simulink library "components_lib"  (Simulink 6.2)
undefined symbols (not defined in the file): A_ang_c, A_att_c, A_est, A_kalman, albedo_onboard_wrapper, B_ang_c, B_att_c, B_est, B_kalman, C_ang_c, C_att_c, C_est, C_i, C_kalman, C_p, Cd, D_ang_c, D_att_c, D_est, D_kalman, Dim, DiscIntNeverNeededParam, Hr, Hs, inerti, Ki, Kr, Ks, magnitude, otoquest, otoquest_with_pro, qmethod, rho, sat_temp_start, ss_proj3, sun_emu_angles2currents, sun_emu_vec2angles, Ts, vector_projection_onto_plane, w_mw_i, w_mw_init, zenith2ref
libraries: components_lib x163, simulink x44, albedo_lib x4, Accessories_lib x3, simulink_extras x2, discrete_bdot_filter x1
(part 4 of 5)

== system components_lib/Orbit and Ephemeris/Orbit and Magnetic field models/SGP4 position ==
  note: Other TLE
  note: Oersted TLE
  JD : Inport  Port=1  LatchInput=off
  Enable : EnablePort
  " S-Function" : S-Function  FunctionName=sgp4S
  Constant : Constant  Value=enable_oersted_tle
  Constant1 : Constant  Value=enable_other_tle
  Demux1 : Demux  Outputs=[3 3]
  Gain 1440 : Gain  Orientation=down  Gain=1440  SaturateOnIntegerOverflow=on
  Mux : Mux  Inputs=2
  Sum : Sum  Orientation=down  Inputs=-+|  SaturateOnIntegerOverflow=on  InputSameDT=on
  Sum1 : Sum  SaturateOnIntegerOverflow=on  InputSameDT=on
  Sum2 : Sum  SaturateOnIntegerOverflow=on  InputSameDT=on
  TLE and time initialization1 : Subsystem  mask{satname='Orsted', YYDDD=02039, JulianDay=2452275.5+40.69255057, xndt2o=0.00002748*0, xndd6o=0, bstar=0.00071190, xincl=96.4788, xnodeo=112.1945, eo=0.0148615, omegao=71.6037, xmo=290.1241, xno=14.43891950, ts=1}
      mask prompts: satname "Satellite Name:"; YYDDD "Epoch [YYDDD]:"; JulianDay "Epoch [JD]:"; xndt2o "MM dot:"; xndd6o "MM dot dot:"; bstar "Drag:"; xincl "Inclination [deg]:"; xnodeo "Right Ascension of Ascending Node [deg]:"; eo "Eccentricity [-]:"; omegao "Argument of Perigee [deg]:"; xmo "Mean Anomaly [deg]:"; xno "Mean Motion [rev/day]:"; ts "Sampling Time [sec]:"
      mask help:
      | Input TLE from the standard Two-Line Orbital Element Set Format
      | Satellite Name, Line 1 and 2.
      mask Display:
      | text(0.35,0.6,'Orbit');
      | text(0.33,0.5,'Model');
      | text(0.3,0.4,'Config');
  TLE and time initialization2 : Subsystem  mask{satname='Orsted', YYDDD=02039, JulianDay=2452275.5+40.69255057, xndt2o=0.00002748*0, xndd6o=0, bstar=0.00071190, xincl=96.4788, xnodeo=112.1945, eo=0.0148615, omegao=71.6037, xmo=290.1241, xno=14.43891950, ts=1}
      mask prompts: satname "Satellite Name:"; YYDDD "Epoch [YYDDD]:"; JulianDay "Epoch [JD]:"; xndt2o "MM dot:"; xndd6o "MM dot dot:"; bstar "Drag:"; xincl "Inclination [deg]:"; xnodeo "Right Ascension of Ascending Node [deg]:"; eo "Eccentricity [-]:"; omegao "Argument of Perigee [deg]:"; xmo "Mean Anomaly [deg]:"; xno "Mean Motion [rev/day]:"; ts "Sampling Time [sec]:"
      mask help:
      | Input TLE from the standard Two-Line Orbital Element Set Format
      | Satellite Name, Line 1 and 2.
      mask Display:
      | text(0.35,0.6,'Orbit');
      | text(0.33,0.5,'Model');
      | text(0.3,0.4,'Config');
  "km -> m" : Gain  Gain=1000  SaturateOnIntegerOverflow=on
  "km/s -> m/s" : Gain  Gain=1000  SaturateOnIntegerOverflow=on
  Position (I) : Outport  InitialOutput=0
  Velocity (I) : Outport  Port=2  InitialOutput=0
  wires:
  [Other_InitJD] -> Sum2/2
  [Oersted_InitJD] -> Sum2/1
  Sum1/1 -> Mux/2
  [Other_TLE] -> Sum1/2
  [Oersted_TLE] -> Sum1/1
  Constant1/1 -> TLE and time initialization2/1(Enable?)
  Constant/1 -> TLE and time initialization1/1(Enable?)
  Gain 1440/1 -> Mux/1
  Sum/1 -> Gain 1440/1
  Sum2/1 -> Sum/1
  Demux1/1 -> "km -> m"/1
  Demux1/2 -> "km/s -> m/s"/1
  " S-Function"/1 -> Demux1/1
  Mux/1 -> " S-Function"/1
  "km/s -> m/s"/1 -> Velocity (I)/1
  "km -> m"/1 -> Position (I)/1
  JD/1 -> Sum/2

== system components_lib/Sensor Emulation/Emulation of gyros/Amplification and ADC ==
  V_cont : Inport  Port=1  LatchInput=off
  Op amp gain [] : Gain  Gain=op_amp_gain
  Quantizer : Quantizer  QuantizationInterval=1/(2^12)
  Sum : Sum  Inputs=|+-
  Sum1 : Sum  Inputs=|++
  op_amp offset [mV] : Constant  Value=op_amp_offset
  V_discrete : Outport
  wires:
  Op amp gain []/1 -> Sum1/1
  Sum/1 -> Op amp gain []/1
  op_amp offset [mV]/1 -> Sum/2, Sum1/2
  V_cont/1 -> Sum/1
  Sum1/1 -> Quantizer/1
  Quantizer/1 -> V_discrete/1

== system components_lib/Sensor Emulation/Emulation of gyros/Gyro sensor block ==
  W(S) [rad/s] : Inport  Port=1  LatchInput=off
  Temperature [K] : Inport  Port=2  LatchInput=off
  Bias [degree/s] : Constant  Value=e_bias
  Drift(offset) [rad/s/K] : Constant  Value=e_drift_offset_model
  Drift(scale factor) [%/K] : Constant  Value=e_drift_scale_model
  "Missalignment correction factor Caculated in mask \"initialization commands\" based on the data supplied in the  missalignment parameter field" : Constant  Value=e_align_coor_factor
  Noise : RandomNumber  Variance=e_noise  Seed=e_noise_seed  SampleTime=0
  Offset  [mV] : Constant  Orientation=up  Value=offset_model
  Product1 : Product  SaturateOnIntegerOverflow=on
  Product2 : Product  Inputs=3  SaturateOnIntegerOverflow=on
  Product3 : Product  SaturateOnIntegerOverflow=on
  Product4 : Product  SaturateOnIntegerOverflow=on
  Scale error [%] : Constant  Value=e_scale
  Sum : Sum  Inputs=|++
  Sum1 : Sum  Inputs=++++++  SaturateOnIntegerOverflow=on
  Sum2 : Sum  Inputs=|+-
  Used for proper  adding of disturbances : Gain  Gain=[1 1 1 -1 -1 -1]
  Used for proper  adding of disturbances1 : Gain  Gain=[1 1 1 -1 -1 -1]
  convert percent to scale factor : Gain  Gain=0.01
  convert percent to scale factor1 : Gain  Gain=0.01
  scale factor : Gain  Gain=scale_model
  temp must be deviation from 25 degree C : Constant  Orientation=up  Value=298.15
  W_sens(S) [mV] : Outport
  wires:
  Noise/1 -> Sum1/4
  Sum1/1 -> Used for proper  adding of disturbances1/1
  W(S) [rad/s]/1 -> Used for proper  adding of disturbances/1
  Product1/1 -> Sum1/1
  Product4/1 -> Sum1/6
  Temperature [K]/1 -> Sum2/1
  temp must be deviation from 25 degree C/1 -> Sum2/2
  Drift(scale factor) [%/K]/1 -> convert percent to scale factor1/1
  Drift(offset) [rad/s/K]/1 -> Product4/2
  convert percent to scale factor1/1 -> Product2/2
  Product2/1 -> Sum1/5
  Bias [degree/s]/1 -> Sum1/3
  convert percent to scale factor/1 -> Product3/1
  Product3/1 -> Sum1/2
  Scale error [%]/1 -> convert percent to scale factor/1
  Used for proper  adding of disturbances/1 -> Product2/1, Product1/2, Product3/2
  "Missalignment correction factor Caculated in mask \"initialization commands\" based on the data supplied in the  missalignment parameter field"/1 -> Product1/1
  Sum2/1 -> Product4/1, Product2/3
  Offset  [mV]/1 -> Sum/2
  Sum/1 -> W_sens(S) [mV]/1
  scale factor/1 -> Sum/1
  Used for proper  adding of disturbances1/1 -> scale factor/1

== system components_lib/Sensor Emulation/Emulation of magnetometer/Amplification and ADC ==
  V_cont : Inport  Port=1  LatchInput=off
  Op amp gain [] : Gain  Gain=op_amp_gain
  Quantizer : Quantizer  QuantizationInterval=1/(2^12)
  Sum1 : Sum  Inputs=|++
  op_amp offset [mV] : Constant  Value=op_amp_offset
  V_discrete : Outport
  wires:
  Quantizer/1 -> V_discrete/1
  Op amp gain []/1 -> Sum1/1
  op_amp offset [mV]/1 -> Sum1/2
  V_cont/1 -> Op amp gain []/1
  Sum1/1 -> Quantizer/1

== system components_lib/Sensor Emulation/Emulation of magnetometer/magnetometer sensor block ==
  B(I) : Inport  Port=1  LatchInput=off
  q(I->S) : Inport  Port=2  LatchInput=off
  Temperature  [K] : Inport  Port=3  LatchInput=off
  Drift(sensitivity) [ppm/K] : Constant  Value=e_drift_sens_model
  "Misalignment correction factor Caculated in mask \"initialization commands\" based on the data supplied in the  misalignment parameter field" : Constant  Value=e_align_coor_factor
  Noise : RandomNumber  Variance=e_noise  Seed=e_noise_seed  SampleTime=0
  Offset  [mV] : Constant  Orientation=up  Value=0
  Scale error : Product  SaturateOnIntegerOverflow=on
  Scale error [%] : Constant  Value=e_scale
  Sensitivity : Gain  Gain=sens_model
  Sum : Sum  Inputs=|++
  Sum1 : Sum  Inputs=++++  SaturateOnIntegerOverflow=on
  Sum2 : Sum  Inputs=|+-
  V*Gauss->Gauss : Gain  Gain=v_supply_model
  Vector rotation by q1 : Subsystem  AncestorBlock=components_lib/Math utilities/Vector operations/Vector rotation by q
  alignment corection  (both orthogonality and  misalignment) : Product  Multiplication=Matrix(*)  SaturateOnIntegerOverflow=on
  convert percent to scale factor : Gain  Gain=0.01
  convert ppm to scale factor : Gain  Gain=10e-6
  sensitivity  temperature  drift [Gauss] : Product  Inputs=3  SaturateOnIntegerOverflow=on
  temp must be deviation from 25 degree C : Constant  Orientation=up  Value=298.15
  Voltage  [mV] : Outport
  wires:
  Sum1/1 -> Sensitivity/1
  Temperature  [K]/1 -> Sum2/1
  temp must be deviation from 25 degree C/1 -> Sum2/2
  q(I->S)/1 -> Vector rotation by q1/1(q)
  "Misalignment correction factor Caculated in mask \"initialization commands\" based on the data supplied in the  misalignment parameter field"/1 -> alignment corection  (both orthogonality and  misalignment)/1
  alignment corection  (both orthogonality and  misalignment)/1 -> sensitivity  temperature  drift [Gauss]/1, Sum1/2, Scale error/2
  Drift(sensitivity) [ppm/K]/1 -> convert ppm to scale factor/1
  convert ppm to scale factor/1 -> sensitivity  temperature  drift [Gauss]/2
  Sum2/1 -> sensitivity  temperature  drift [Gauss]/3
  Vector rotation by q1/1(q'Vq) -> alignment corection  (both orthogonality and  misalignment)/2  "B(S)"
  Sum/1 -> Voltage  [mV]/1
  Sensitivity/1 -> V*Gauss->Gauss/1
  Offset  [mV]/1 -> Sum/2
  V*Gauss->Gauss/1 -> Sum/1
  B(I)/1 -> Vector rotation by q1/2(V)
  sensitivity  temperature  drift [Gauss]/1 -> Sum1/3
  convert percent to scale factor/1 -> Scale error/1
  Scale error/1 -> Sum1/1
  Scale error [%]/1 -> convert percent to scale factor/1
  Noise/1 -> Sum1/4

== system components_lib/Sensor Emulation/Sun sensors/Amplification and ADC ==
  Currents [mA] : Inport  Port=1  LatchInput=off
  Op amp gain : Gain  Gain=op_amp_gain
  Quantizer : Quantizer  QuantizationInterval=1/(2^12)
  Sum1 : Sum  Inputs=|++
  op_amp offset [mV] : Constant  Value=op_amp_offset
  I_ADC [mA] : Outport
  wires:
  Sum1/1 -> Quantizer/1
  Quantizer/1 -> I_ADC [mA]/1
  Op amp gain/1 -> Sum1/1
  op_amp offset [mV]/1 -> Sum1/2
  Currents [mA]/1 -> Op amp gain/1

== system components_lib/Sensor Emulation/Sun sensors/Frame conversion ==
  note: Sun vector
      | from sun to sat
      | in ECI
  Sun pos. R_s(I) : Inport  Port=1  LatchInput=off
  S/C pos. R_sa(I) : Inport  Port=2  LatchInput=off
  q(I->S) : Inport  Port=3  LatchInput=off
  q(I->E) : Inport  Port=4  LatchInput=off
  Quaternion inverter : components_lib/Math utilities/Quaternion operations/Quaternion inverter
  Rotation of q1 by q2 : components_lib/Math utilities/Quaternion operations/Rotation of q1 by q2
  Sum : Sum  Inputs=|+-
  Vector rotation by q : components_lib/Math utilities/Quaternion operations/Vector rotation by q
  Vector rotation by q3 : components_lib/Math utilities/Quaternion operations/Vector rotation by q
  "Zenith to nadir " : Gain  Gain=-1
  Sun pos. R_s(S) : Outport
  Nadir(E) : Outport  Port=2
  q(S->E) : Outport  Port=3
  wires:
  Sum/1 -> Vector rotation by q3/2
  Sun pos. R_s(I)/1 -> Sum/1
  Rotation of q1 by q2/1 -> q(S->E)/1
  Quaternion inverter/1 -> Rotation of q1 by q2/1
  q(I->S)/1 -> Quaternion inverter/1, Vector rotation by q3/1
  q(I->E)/1 -> Rotation of q1 by q2/2, Vector rotation by q/1
  "Zenith to nadir "/1 -> Nadir(E)/1
  S/C pos. R_sa(I)/1 -> Sum/2, Vector rotation by q/2
  Vector rotation by q/1 -> "Zenith to nadir "/1
  Vector rotation by q3/1 -> Sun pos. R_s(S)/1

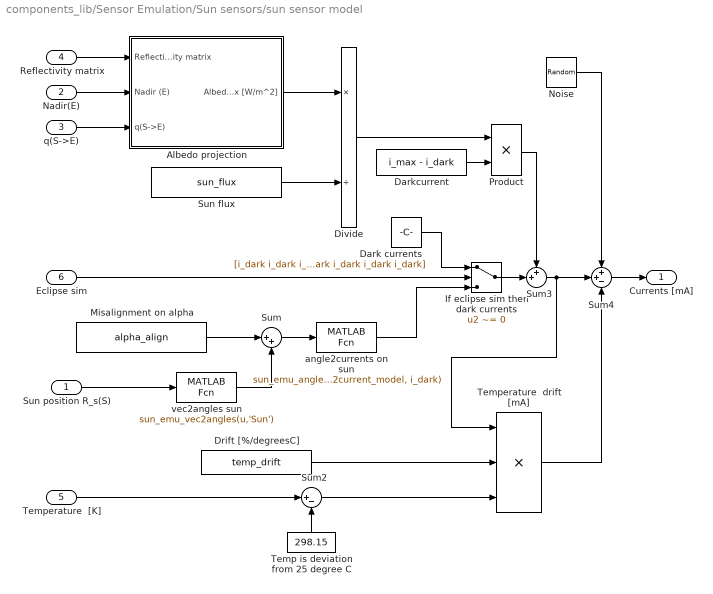
== system components_lib/Sensor Emulation/Sun sensors/sun sensor model ==
  Sun position R_s(S) : Inport  Port=1  LatchInput=off
  Nadir(E) : Inport  Port=2  LatchInput=off
  q(S->E) : Inport  Port=3  LatchInput=off
  Reflectivity matrix : Inport  Port=4  LatchInput=off
  Temperature  [K] : Inport  Port=5  LatchInput=off
  Eclipse sim : Inport  Port=6  PortDimensions=1  LatchInput=off
  Albedo projection : Subsystem
  Dark currents : Constant  Value=[i_dark i_dark i_dark i_dark i_dark i_dark]
  Darkcurrent : Constant  Value=i_max - i_dark
  Divide : Product  Inputs=*/  OutScaling=2^-10
  Drift [%/degreesC] : Constant  Value=temp_drift
  If eclipse sim then dark currents : Switch  Criteria=u2 ~= 0
  Misalignment on alpha : Constant  Value=alpha_align
  Noise : RandomNumber  Variance=sigma_noise^2  Seed=noise_seed  SampleTime=0
  Product : Product  RndMeth=Zero
  Sum : Sum  Inputs=|++
  Sum2 : Sum  Inputs=|+-
  Sum3 : Sum  Inputs=++|
  Sum4 : Sum  Inputs=++-
  Sun flux : Constant  Value=sun_flux
  Temp is deviation from 25 degree C : Constant  Orientation=up  Value=298.15
  Temperature  drift [mA] : Product  Inputs=3  SaturateOnIntegerOverflow=on
  angle2currents on sun : MATLABFcn  MATLABFcn=sun_emu_angles2currents(u,angle2current_model, i_dark)
  vec2angles sun : MATLABFcn  MATLABFcn=sun_emu_vec2angles(u,'Sun')
  Currents [mA] : Outport
  wires:
  If eclipse sim then dark currents/1 -> Sum3/2
  angle2currents on sun/1 -> If eclipse sim then dark currents/3
  Eclipse sim/1 -> If eclipse sim then dark currents/2
  Dark currents/1 -> If eclipse sim then dark currents/1
  Sum4/1 -> Currents [mA]/1
  Temperature  drift [mA]/1 -> Sum4/3
  Sum3/1 -> Sum4/2, Temperature  drift [mA]/1
  Product/1 -> Sum3/1
  Temperature  [K]/1 -> Sum2/1
  Noise/1 -> Sum4/1
  Albedo projection/1(Albedo flux [W/m^2]) -> Divide/1
  Nadir(E)/1 -> Albedo projection/2(Nadir (E))
  q(S->E)/1 -> Albedo projection/3(q(S->E))
  Reflectivity matrix/1 -> Albedo projection/1(Reflectivity matrix)
  Darkcurrent/1 -> Product/2
  Temp is deviation from 25 degree C/1 -> Sum2/2
  Misalignment on alpha/1 -> Sum/1
  vec2angles sun/1 -> Sum/2
  Sum/1 -> angle2currents on sun/1
  Sum2/1 -> Temperature  drift [mA]/3
  Drift [%/degreesC]/1 -> Temperature  drift [mA]/2
  Sun position R_s(S)/1 -> vec2angles sun/1
  Sun flux/1 -> Divide/2
  Divide/1 -> Product/1

== system components_lib/ACS/Controllers/Desaturation controller/Trigger ==
  B_unit(s) : Inport  Port=1  PortDimensions=3  LatchInput=off
  h_err : Inport  Port=2  LatchInput=off
  Dot Product2 : simulink/Math Operations/Dot Product  InputSameDT=on  OutDataType=sfix(16)  OutScaling=2^-10  DoSatur=off
  Dot Product3 : simulink/Math Operations/Dot Product  InputSameDT=on  OutDataType=sfix(16)  OutScaling=2^-10  DoSatur=off
  Math Function1 : Math  Operator=sqrt  SaturateOnIntegerOverflow=on
  Math Function3 : Math  Operator=sqrt  SaturateOnIntegerOverflow=on
  Relay : Subsystem
  Saturation : Saturate  UpperLimit=inf  LowerLimit=2*sin(deg2rad(2))*h_bias
  Sum1 : Sum  Inputs=|+-
  angular momentum bias1 : Constant  Value=sin(deg2rad(2))*h_bias
  angular momentum bias3 : Constant  Value=2*5.48e-5
  angular momentum bias4 : Constant  Value=h_bias
  cross_product : components_lib/Math utilities/Vector operations/cross_product_no_fnc
  mag B div1 : Product  Inputs=*/  OutScaling=2^-10
  mg B div4 : Product  OutScaling=2^-10
  switch : Outport
  wires:
  angular momentum bias3/1 -> Sum1/2
  Relay/1(Switch) -> switch/1
  angular momentum bias4/1 -> mg B div4/2
  mg B div4/1 -> Sum1/1
  Dot Product2/1 -> Math Function3/1
  Dot Product3/1 -> Math Function1/1
  Math Function1/1 -> mag B div1/2
  Sum1/1 -> Saturation/1
  mag B div1/1 -> mg B div4/1  "sin(a)"
  h_err/1 -> Dot Product3/1, Dot Product3/2, cross_product/1
  B_unit(s)/1 -> cross_product/2
  cross_product/1 -> Dot Product2/1, Dot Product2/2
  Math Function3/1 -> mag B div1/1, Relay/1(||Herr x B_unit||)
  angular momentum bias1/1 -> Relay/3(lower limet)
  Saturation/1 -> Relay/2(upper limet)

== system components_lib/ACS/Controllers/Desaturation controller/m_mt to v_mt conversion ==
  m_mt : Inport  Port=1  LatchInput=off
  T_meas : Inport  Port=2  LatchInput=off
  Demux : Demux  Outputs=3
  Gain : Gain  Gain=1/(n_mt(1)*A_mt(1))
  Gain1 : Gain  Gain=1/(n_mt(2)*A_mt(2))
  Gain2 : Gain  Gain=1/(n_mt(3)*A_mt(3))
  Mux : Mux  Inputs=3
  Resistance for mt on x-axis : Subsystem  mask{A_wire_mt=(pi/4)*0.0002^2, sigma_0_mt=1.7e-8, alpha_0_mt=3.9e-3, T_0_mt=293}
      mask prompts: A_wire_mt "Wire cross sectional area"; sigma_0_mt "Wire resistivity"; alpha_0_mt "Wire resistivity temp. coef."; T_0_mt "Wire resistivity base temp."
  Resistance for mt on y-axis : Subsystem  mask{A_wire_mt=(pi/4)*0.0002^2, sigma_0_mt=1.7e-8, alpha_0_mt=3.9e-3, T_0_mt=293}
      mask prompts: A_wire_mt "Wire cross sectional area"; sigma_0_mt "Wire resistivity"; alpha_0_mt "Wire resistivity temp. coef."; T_0_mt "Wire resistivity base temp."
  Resistance for mt on z-axis : Subsystem  mask{A_wire_mt=(pi/4)*0.0002^2, sigma_0_mt=1.7e-8, alpha_0_mt=3.9e-3, T_0_mt=293}
      mask prompts: A_wire_mt "Wire cross sectional area"; sigma_0_mt "Wire resistivity"; alpha_0_mt "Wire resistivity temp. coef."; T_0_mt "Wire resistivity base temp."
  electromechanis transfer funtion for mt_x : Subsystem
  "electromechanis transfer funtion for mt_y " : Subsystem
  "electromechanis transfer funtion for mt_z " : Subsystem
  i_mt : Scope  NumInputPorts=3
      settings: YMin=-5~-5~-5  YMax=5~5~5  SaveName=ScopeData8
  v_mt : Outport
  wires:
  Demux/3 -> Gain2/1
  Demux/2 -> Gain1/1
  Demux/1 -> Gain/1
  Gain/1 -> electromechanis transfer funtion for mt_x/1(i_mt), i_mt/1
  Gain1/1 -> "electromechanis transfer funtion for mt_y "/1(i_mt), i_mt/2
  Gain2/1 -> "electromechanis transfer funtion for mt_z "/1(i_mt), i_mt/3
  m_mt/1 -> Demux/1
  "electromechanis transfer funtion for mt_y "/1(v_mt) -> Mux/2
  "electromechanis transfer funtion for mt_z "/1(v_mt) -> Mux/3
  Resistance for mt on x-axis/1(R(T)) -> electromechanis transfer funtion for mt_x/2(R(T))
  Resistance for mt on y-axis/1(R(T)) -> "electromechanis transfer funtion for mt_y "/2(R(T))
  Resistance for mt on z-axis/1(R(T)) -> "electromechanis transfer funtion for mt_z "/2(R(T))
  T_meas/1 -> Resistance for mt on y-axis/1(T), Resistance for mt on x-axis/1(T), Resistance for mt on z-axis/1(T)
  electromechanis transfer funtion for mt_x/1(v_mt) -> Mux/1
  Mux/1 -> v_mt/1

== system components_lib/ACS/Controllers/Detumble controller/Continous B-dot controller ==
  B(S) : Inport  Port=1  LatchInput=off
  Gain : Gain  Gain=w_c
  Gain1 : Gain  Gain=-C_cont
  Integrator : Integrator  Orientation=left
  Sum : Sum  Inputs=|+-
  m_mt(S) : Outport
  wires:
  B(S)/1 -> Sum/1
  Sum/1 -> Gain/1
  Gain/1 -> Gain1/1, Integrator/1
  Integrator/1 -> Sum/2
  Gain1/1 -> m_mt(S)/1

== system components_lib/ACS/Controllers/Detumble controller/Discrete B-dot controller ==
  B(S) : Inport  Port=1  LatchInput=off
  Clock : Clock
  Discrete B-dot filter : discrete_bdot_filter/Discrete B-dot filter
  Gain1 : Gain  Gain=-C_disc
  If : If  IfExpression=u1 > 2
  If1 : If  IfExpression=u1 < 4
  If2 : If  IfExpression=u1 < 2
  Subsystem1 : Subsystem  AncestorBlock=attitude_control_lib/Attitude Control/B-dot controller disc/Subsystem2
  Subsystem2 : Subsystem  AncestorBlock=attitude_control_lib/Attitude Control/B-dot controller disc/Subsystem2
  Subsystem3 : Subsystem  AncestorBlock=attitude_control_lib/Attitude Control/B-dot controller disc/Subsystem2
  mod 10 : MATLABFcn  MATLABFcn=mod(u(1),4)
  m_mt(s) : Outport
  wires:
  Discrete B-dot filter/1 -> Gain1/1
  If1/1 -> Subsystem3/Action
  Subsystem2/1(Out1) -> m_mt(s)/1
  B(S)/1 -> Subsystem1/1(In1)
  Subsystem3/1(Out1) -> Subsystem2/1(In1)
  Gain1/1 -> Subsystem3/1(In1)
  Subsystem1/1(Out1) -> Discrete B-dot filter/1
  Clock/1 -> mod 10/1
  mod 10/1 -> If2/1, If1/1, If/1
  If2/1 -> Subsystem1/Action
  If/1 -> Subsystem2/Action

== system components_lib/ACS/Controllers/Detumble controller/Magnetic field I to S ==
  q(I->S) : Inport  Port=1  LatchInput=off
  B(I) : Inport  Port=2  LatchInput=off
  Gauss to Tesla : Gain  Gain=1e-4
  Vector rotation by q1 : components_lib/Math utilities/Quaternion operations/Vector rotation by q
  B(S) : Outport
  wires:
  B(I)/1 -> Vector rotation by q1/2
  Gauss to Tesla/1 -> B(S)/1
  Vector rotation by q1/1 -> Gauss to Tesla/1
  q(I->S)/1 -> Vector rotation by q1/1

== system components_lib/ACS/Controllers/Detumble controller/enable/disable continous controller ==
  In1 : Inport  Port=1  LatchInput=off
  Action Port : ActionPort
  Out1 : Outport
  wires:
  In1/1 -> Out1/1

== system components_lib/ACS/Controllers/Detumble controller/enable/disable discrete controller ==
  In1 : Inport  Port=1  LatchInput=off
  Action Port : ActionPort
  Out1 : Outport
  wires:
  In1/1 -> Out1/1

== system components_lib/ADS/On-board model/ADS on-board models/Albedo model onboard ==
  "Earth -> Sun vector (ECEF)" : Inport  Port=1  LatchInput=off
  Zenith vector (ECEF) : Inport  Port=2  LatchInput=off
  q(I->S) : Inport  Port=3  LatchInput=off
  q(I->E) : Inport  Port=4  LatchInput=off
  On : Constant  Orientation=down  Value=enable
  On1 : Constant  Orientation=down  Value=~enable
  Sum : Sum  Inputs=|++
  cos dependent albedo : Subsystem
  fov matrix albedo : Subsystem
  Albedo vector (I) : Outport
  wires:
  On1/1 -> cos dependent albedo/Enable
  fov matrix albedo/1(Albedo vector (I)) -> Sum/2
  cos dependent albedo/1(Albedo vector (I)) -> Sum/1
  On/1 -> fov matrix albedo/Enable
  Zenith vector (ECEF)/1 -> fov matrix albedo/1(Zenith vector (ECEF)), cos dependent albedo/2(Zenith vector (ECEF))
  "Earth -> Sun vector (ECEF)"/1 -> fov matrix albedo/2("Earth -> Sun vector (ECEF)"), cos dependent albedo/1("Earth -> Sun vector (ECEF)")
  q(I->E)/1 -> fov matrix albedo/4(q(I->E))
  q(I->S)/1 -> fov matrix albedo/3(q(I->S))
  Sum/1 -> Albedo vector (I)/1

== system components_lib/ADS/On-board model/Albedo model onboard/cos dependent albedo ==
  note: Projection onto
      | the zenith vector
  "Earth -> Sun vector (ECEF)" : Inport  Port=1  LatchInput=off
  Zenith vector (ECEF) : Inport  Port=2  LatchInput=off
  Enable : EnablePort  StatesWhenEnabling=reset
  Abs : Abs
  Dot Product : simulink/Math Operations/Dot Product  InputSameDT=on  OutDataType=sfix(16)  OutScaling=2^-10  DoSatur=off
  Mean solar flux (1366.9 [W/m^2]) : Constant  Value=sun_flux
  Product : Product  RndMeth=Zero
  Product1 : Product  RndMeth=Zero
  Product2 : Product  RndMeth=Zero
  Sun vector  to unit vector : components_lib/Math utilities/Vector operations/to unit vector
  Zentih vector to unit vector : components_lib/Math utilities/Vector operations/to unit vector
  "zenith2ref(u, mrm)" : MATLABFcn  MATLABFcn=zenith2ref(u, mrm)*2
  Albedo vector (I) : Outport
  wires:
  Product2/1 -> Albedo vector (I)/1
  Product1/1 -> Product2/1
  Abs/1 -> Product1/1
  Dot Product/1 -> Abs/1
  Sun vector  to unit vector/1 -> Product/1
  Mean solar flux (1366.9 [W/m^2])/1 -> Product/2
  Product/1 -> Dot Product/1
  "zenith2ref(u, mrm)"/1 -> Product1/2
  Zentih vector to unit vector/1 -> Product2/2, "zenith2ref(u, mrm)"/1, Dot Product/2
  "Earth -> Sun vector (ECEF)"/1 -> Sun vector  to unit vector/1
  Zenith vector (ECEF)/1 -> Zentih vector to unit vector/1

== system components_lib/ADS/On-board model/Albedo model onboard/fov matrix albedo ==
  Zenith vector (ECEF) : Inport  Port=1  LatchInput=off
  "Earth -> Sun vector (ECEF)" : Inport  Port=2  LatchInput=off
  q(I->S) : Inport  Port=3  LatchInput=off
  q(I->E) : Inport  Port=4  LatchInput=off
  Enable : EnablePort  StatesWhenEnabling=reset
  Albedo projection : components_lib/ADS/On-board Sensor model/Albedo projection
  Demux : Demux  Outputs=2
  Earth Albedo Model : Subsystem  TreatAsAtomicUnit=on  mask(Earth Albedo Model){eprdata=load('lib/space_environment_emulation/albedo/toolbox/epr_data/2003/ga030101-031231'), redfac=10, Ts=1, enable=on}
      mask prompts: eprdata "Reflectivity Data (EPR Struct):"; redfac "Reduction factor:"; Ts "Sample Time (-1 for inherited):"
      mask help: Calculate Earth Albedo using static data from the EP/TOMS spacecraft.
      mask init:
      | global sy;
      | global sx;
      | sy = round(180/redfac);
      | sx = round(288/redfac);
      mask Help:
      | <b>Input</b><br>
      | Sat: Vector to satellite in ECEF [m]<br>
      | Sun: Vector to the Sun in ECEF [m]<p>
      | <b>Parameters</b><br>
      | Reflectivity Data (EPR Struct): TOMS Reflectivity data [E.U].<br>
      | Reduction factor: Reduce data resolution by this factor.<br>
      | Sample Time (-1 for inherited): Sample Time [s]. The block cannot inherit continuous sample time.<br>
      | Enable: Enable or disable albedo calculation<p>
      | <b>Output</b><br>
      | Albedo: Fraction of solar irradiance received on the satellite. The incoming solar irradiance is 1366.5 W/m^2<p>
      mask CallbackString: |||enable = strcmp(get_param(gcb,'enable'),'on');
      mask Display:
      | image(imread('private/albedoicon.png'));
      | port_label('output', 1, 'Albedo');
      | port_label('input', 1, 'Sat');
      | port_label('input', 2, 'Sun');
  Quaternion inverter1 : components_lib/Math utilities/Quaternion operations/Quaternion inverter
  Rotation of q1 by q2 : components_lib/Math utilities/Quaternion operations/Rotation of q1 by q2
  Sum : Sum  Inputs=|+-
  Vector rotation by q4 : components_lib/Math utilities/Quaternion operations/Vector rotation by q
  "Zenith to nadir " : Gain  Gain=-1
  Albedo vector (I) : Outport
  wires:
  "Earth -> Sun vector (ECEF)"/1 -> Earth Albedo Model/2(r_sun_ecef)
  Zenith vector (ECEF)/1 -> "Zenith to nadir "/1, Earth Albedo Model/1(r_sat_ecef)
  Vector rotation by q4/1 -> Albedo vector (I)/1
  q(I->E)/1 -> Rotation of q1 by q2/2
  q(I->S)/1 -> Quaternion inverter1/1
  Earth Albedo Model/1(a) -> Albedo projection/1
  "Zenith to nadir "/1 -> Albedo projection/2
  Quaternion inverter1/1 -> Rotation of q1 by q2/1, Vector rotation by q4/1
  Rotation of q1 by q2/1 -> Albedo projection/3
  Albedo projection/1 -> Demux/1
  Demux/1 -> Sum/1
  Demux/2 -> Sum/2
  Sum/1 -> Vector rotation by q4/2

== system components_lib/ADS/On-board model/Ephemeris on-board/ECEF ==
  t(JD) : Inport  Port=1  LatchInput=off
  eci2ecef : MATLABFcn  MATLABFcn=eci2ecef  OutputDimensions=4
  q(I->E) : Outport
  wires:
  eci2ecef/1 -> q(I->E)/1
  t(JD)/1 -> eci2ecef/1

== system components_lib/ADS/On-board model/Ephemeris on-board/Sun Position ==
  t(JD) : Inport  Port=1  LatchInput=off
  Sun R in ECI : MATLABFcn  MATLABFcn=sun  OutputDimensions=3
  R_s(I) : Outport
  wires:
  t(JD)/1 -> Sun R in ECI/1
  Sun R in ECI/1 -> R_s(I)/1

== system components_lib/ADS/On-board model/Gyros/Combine the angular rate  from the 6 gyros to angular  rate in S-frame ==
  W_meas 6 gyros : Inport  Port=1  LatchInput=off
  Demux : Demux  Outputs=6
  Gain1 : Gain  Gain=0.5
  Mux : Mux  Inputs=3
  Sum : Sum  Inputs=|+-
  Sum5 : Sum  Inputs=|+-
  Sum6 : Sum  Inputs=|+-
  W_meas (S) : Outport
  wires:
  Gain1/1 -> W_meas (S)/1
  W_meas 6 gyros/1 -> Demux/1
  Mux/1 -> Gain1/1
  Sum6/1 -> Mux/3
  Sum5/1 -> Mux/2
  Sum/1 -> Mux/1
  Demux/6 -> Sum6/2
  Demux/3 -> Sum6/1
  Demux/5 -> Sum5/2
  Demux/2 -> Sum5/1
  Demux/4 -> Sum/2
  Demux/1 -> Sum/1

== system components_lib/ADS/On-board model/Orbit and Magnetic field models/TLE and time initialization1 ==
  Enable? : Inport  Port=1  LatchInput=off
  Create TLE and JD : Subsystem  TreatAsAtomicUnit=on
  Oersted_InitJD : Outport
  Oersted_TLE : Outport  Port=2
  wires:
  Enable?/1 -> Create TLE and JD/Enable
  Create TLE and JD/2("TLE ") -> Oersted_TLE/1
  Create TLE and JD/1(Init JD) -> Oersted_InitJD/1

== system components_lib/ADS/On-board model/Orbit and Magnetic field models/TLE and time initialization3 ==
  Enable? : Inport  Port=1  LatchInput=off
  Create TLE and JD : Subsystem  TreatAsAtomicUnit=on
  Other_InitJD : Outport
  Other_TLE : Outport  Port=2
  wires:
  Enable?/1 -> Create TLE and JD/Enable
  Create TLE and JD/2("TLE ") -> Other_TLE/1
  Create TLE and JD/1(Init JD) -> Other_InitJD/1

== system components_lib/Disturbances/Exposed area/Shadow Area/Subsystem ==
  x : Inport  Port=1  LatchInput=off
  Dot Product13 : simulink/Math Operations/Dot Product  InputSameDT=on  OutDataType=sfix(16)  OutScaling=2^-10  DoSatur=off
  inv9 : Math  Operator=sqrt  SaturateOnIntegerOverflow=on
  norm(x) : Outport
  wires:
  inv9/1 -> norm(x)/1
  Dot Product13/1 -> inv9/1
  x/1 -> Dot Product13/2, Dot Product13/1  "pxp"

== system components_lib/Disturbances/Exposed area/Shadow Area/Subsystem1 ==
  x : Inport  Port=1  LatchInput=off
  Dot Product13 : simulink/Math Operations/Dot Product  InputSameDT=on  OutDataType=sfix(16)  OutScaling=2^-10  DoSatur=off
  inv9 : Math  Operator=sqrt  SaturateOnIntegerOverflow=on
  norm(x) : Outport
  wires:
  x/1 -> Dot Product13/1, Dot Product13/2  "pxp"
  Dot Product13/1 -> inv9/1
  inv9/1 -> norm(x)/1

== system components_lib/Disturbances/Exposed area/Shadow Area/Subsystem2 ==
  x : Inport  Port=1  LatchInput=off
  Dot Product13 : simulink/Math Operations/Dot Product  InputSameDT=on  OutDataType=sfix(16)  OutScaling=2^-10  DoSatur=off
  inv9 : Math  Operator=sqrt  SaturateOnIntegerOverflow=on
  norm(x) : Outport
  wires:
  inv9/1 -> norm(x)/1
  Dot Product13/1 -> inv9/1
  x/1 -> Dot Product13/2, Dot Product13/1  "pxp"

== system components_lib/Disturbances/Exposed area/Shadow Area/Subsystem3 ==
  x : Inport  Port=1  LatchInput=off
  Dot Product13 : simulink/Math Operations/Dot Product  InputSameDT=on  OutDataType=sfix(16)  OutScaling=2^-10  DoSatur=off
  inv9 : Math  Operator=sqrt  SaturateOnIntegerOverflow=on
  norm(x) : Outport
  wires:
  inv9/1 -> norm(x)/1
  Dot Product13/1 -> inv9/1
  x/1 -> Dot Product13/2, Dot Product13/1  "pxp"

== system components_lib/Disturbances/Gravity/Gravity Gradient Torque/  ==
  q(C->SC) : Inport  Port=1  LatchInput=off
  "q(I -> SC)" : Inport  Port=2  LatchInput=off
  R_sc(I) : Inport  Port=3  LatchInput=off
  Reverse quaternion rotation : components_lib/Math utilities/Quaternion operations/Reverse quaternion rotation
  Rotation of q1 by q2 : components_lib/Math utilities/Quaternion operations/Rotation of q1 by q2
  Vector rotation by q : components_lib/Math utilities/Quaternion operations/Vector rotation by q
  to unit vector : components_lib/Math utilities/Vector operations/to unit vector
  R_sc(C) : Outport
  wires:
  Vector rotation by q/1 -> R_sc(C)/1
  to unit vector/1 -> Vector rotation by q/2
  Rotation of q1 by q2/1 -> Vector rotation by q/1
  R_sc(I)/1 -> to unit vector/1
  Reverse quaternion rotation/1 -> Rotation of q1 by q2/2
  q(C->SC)/1 -> Reverse quaternion rotation/1
  "q(I -> SC)"/1 -> Rotation of q1 by q2/1

== system components_lib/Math utilities/Quaternion operations/Reverse quaternion rotation/Quaternion inverter ==
  q : Inport  Port=1  LatchInput=off
  Demux : Demux
  Demux1 : Demux  Outputs=3
  Gain : Gain  Gain=-1  SaturateOnIntegerOverflow=on
  Mux : Mux
  Mux1 : Mux  Inputs=3
  q^-1 : Outport
  wires:
  Gain/1 -> Demux1/1
  Demux1/3 -> Mux/3
  Demux1/2 -> Mux/2
  Demux1/1 -> Mux/1
  Mux1/1 -> Gain/1
  Demux/3 -> Mux1/3
  Demux/2 -> Mux1/2
  Demux/1 -> Mux1/1
  Demux/4 -> Mux/4
  Mux/1 -> q^-1/1
  q/1 -> Demux/1

== system components_lib/Math utilities/Quaternion operations/Vector rotation by q/Quaternion inverter ==
  q : Inport  Port=1  LatchInput=off
  Demux : Demux
  Demux1 : Demux  Outputs=3
  Gain : Gain  Gain=-1  SaturateOnIntegerOverflow=on
  Mux : Mux
  Mux1 : Mux  Inputs=3
  q^-1 : Outport
  wires:
  Gain/1 -> Demux1/1
  Demux1/3 -> Mux/3
  Demux1/2 -> Mux/2
  Demux1/1 -> Mux/1
  Mux1/1 -> Gain/1
  Demux/3 -> Mux1/3
  Demux/2 -> Mux1/2
  Demux/1 -> Mux1/1
  Demux/4 -> Mux/4
  Mux/1 -> q^-1/1
  q/1 -> Demux/1

== system components_lib/Math utilities/Vector operations/Vector rotation by q/Quaternion inverter ==
  q : Inport  Port=1  LatchInput=off
  Demux : Demux
  Demux1 : Demux  Outputs=3
  Gain : Gain  Gain=-1  SaturateOnIntegerOverflow=on
  Mux : Mux
  Mux1 : Mux  Inputs=3
  q^-1 : Outport
  wires:
  Gain/1 -> Demux1/1
  Demux1/3 -> Mux/3
  Demux1/2 -> Mux/2
  Demux1/1 -> Mux/1
  Mux1/1 -> Gain/1
  Demux/3 -> Mux1/3
  Demux/2 -> Mux1/2
  Demux/1 -> Mux1/1
  Demux/4 -> Mux/4
  Mux/1 -> q^-1/1
  q/1 -> Demux/1

== system components_lib/Orbit and Ephemeris/Orbit and Magnetic field models/Oersted time/JD and sec. to Julian Date ==
  Second of Day : Inport  Port=1  LatchInput=off
  Day as Julian Date : Inport  Port=2  LatchInput=off
  Calc. TimeString : S-Function  FunctionName=Qcontinuum
  Sec2Day : Gain  Gain=1/86400  SaturateOnIntegerOverflow=on
  Sum : Sum  Inputs=++|  SaturateOnIntegerOverflow=on  InputSameDT=on
  Julian Date (Day) : Outport
  wires:
  Calc. TimeString/1 -> Sec2Day/1
  Sec2Day/1 -> Sum/1
  Day as Julian Date/1 -> Sum/2
  Second of Day/1 -> Calc. TimeString/1
  Sum/1 -> Julian Date (Day)/1

== system components_lib/Orbit and Ephemeris/Orbit and Magnetic field models/SGP4 position/TLE and time initialization1 ==
  Enable? : Inport  Port=1  LatchInput=off
  Create TLE and JD : Subsystem  TreatAsAtomicUnit=on
  tag scope: Oersted_InitJD=global, Oersted_TLE=global
  wires:
  Enable?/1 -> Create TLE and JD/Enable
  Create TLE and JD/2("TLE ") -> [Oersted_TLE]
  Create TLE and JD/1(Init JD) -> [Oersted_InitJD]

== system components_lib/Orbit and Ephemeris/Orbit and Magnetic field models/SGP4 position/TLE and time initialization2 ==
  Enable? : Inport  Port=1  LatchInput=off
  Create TLE and JD : Subsystem  TreatAsAtomicUnit=on
  tag scope: Other_InitJD=global, Other_TLE=global
  wires:
  Create TLE and JD/1(Init JD) -> [Other_InitJD]
  Create TLE and JD/2("TLE ") -> [Other_TLE]
  Enable?/1 -> Create TLE and JD/Enable

== system components_lib/Sensor Emulation/Emulation of magnetometer/magnetometer sensor block/Vector rotation by q1 ==
  q : Inport  Port=1  LatchInput=off
  V : Inport  Port=2  LatchInput=off
  Constant : Constant  Value=0
  Demux : Demux  Outputs=3
  Demux1 : Demux
  Mux : Mux
  Mux1 : Mux  Inputs=3
  Quaternion inverter : Subsystem
  Quaternion mulitiplication : S-Function  FunctionName=qmul
  Quaternion mulitiplication1 : S-Function  FunctionName=qmul
  Terminator : Terminator
  q'Vq : Outport
  wires:
  Mux1/1 -> q'Vq/1
  Demux1/4 -> Terminator/1
  Demux1/3 -> Mux1/3
  Demux1/2 -> Mux1/2
  Demux1/1 -> Mux1/1
  Quaternion mulitiplication1/1 -> Demux1/1
  Quaternion mulitiplication/1 -> Quaternion mulitiplication1/1
  Mux/1 -> Quaternion mulitiplication/2
  Constant/1 -> Mux/4
  Demux/3 -> Mux/3
  Demux/2 -> Mux/2
  Demux/1 -> Mux/1
  V/1 -> Demux/1
  Quaternion inverter/1(q^-1) -> Quaternion mulitiplication/1
  q/1 -> Quaternion mulitiplication1/2, Quaternion inverter/1(q)

== system components_lib/Sensor Emulation/Sun sensors/sun sensor model/Albedo projection ==
  Reflectivity matrix : Inport  Port=1  LatchInput=off
  Nadir (E) : Inport  Port=2  LatchInput=off
  q(S->E) : Inport  Port=3  LatchInput=off
  Mux7 : Mux
  Reshape : simulink/Math Operations/Reshape  OutputDimensionality=1-D array  OutputDimensions=[1,1]
  Vector rotation by q : components_lib/Math utilities/Quaternion operations/Vector rotation by q
  Vector rotation by q1 : components_lib/Math utilities/Quaternion operations/Vector rotation by q
  X+ vector (SC) : Constant  Value=[1 0 0]
  ss_proj : MATLABFcn  MATLABFcn=ss_proj3(u(length(u)-8:length(u)-6),u(length(u)-5:length(u)-3),u(length(u)-2:length(u)),reshape(u(1:length(u)-9),round([180,288]/sqrt(51840/(length(u)-9)))))
  y+ vector (SC) : Constant  Value=[0 1 0]
  Albedo flux [W/m^2] : Outport
  wires:
  ss_proj/1 -> Albedo flux [W/m^2]/1
  Mux7/1 -> ss_proj/1
  Reshape/1 -> Mux7/1
  Vector rotation by q/1 -> Mux7/3
  Vector rotation by q1/1 -> Mux7/4
  y+ vector (SC)/1 -> Vector rotation by q1/2
  X+ vector (SC)/1 -> Vector rotation by q/2
  q(S->E)/1 -> Vector rotation by q1/1, Vector rotation by q/1
  Nadir (E)/1 -> Mux7/2  "nadir"
  Reflectivity matrix/1 -> Reshape/1

== system components_lib/ACS/Controllers/Desaturation controller/Trigger/Relay ==
  ||Herr x B_unit|| : Inport  Orientation=down  Port=1  LatchInput=off
  upper limet : Inport  Port=2  LatchInput=off
  lower limet : Inport  Port=3  LatchInput=off
  Logical Operator1 : Logic  AllPortsSameDT=off  OutDataTypeMode=Boolean
  Logical Operator2 : Logic  Operator=OR  AllPortsSameDT=off  OutDataTypeMode=Boolean
  Logical Operator3 : Logic  AllPortsSameDT=off  OutDataTypeMode=Boolean
  Memory : Memory  Orientation=left
  Relational Operator : RelationalOperator  Operator=>  LogicOutDataTypeMode=Boolean  LogicDataType=1
  Relational Operator1 : RelationalOperator  Operator=>  LogicOutDataTypeMode=Boolean  LogicDataType=1
  Switch : Outport
  wires:
  ||Herr x B_unit||/1 -> Relational Operator/1, Relational Operator1/1
  Relational Operator1/1 -> Logical Operator1/1, Logical Operator3/2
  Logical Operator1/1 -> Logical Operator2/2
  Logical Operator2/1 -> Memory/1, Switch/1
  Memory/1 -> Logical Operator1/2
  upper limet/1 -> Relational Operator/2
  lower limet/1 -> Relational Operator1/2
  Relational Operator/1 -> Logical Operator3/1
  Logical Operator3/1 -> Logical Operator2/1

== system components_lib/ACS/Controllers/Desaturation controller/m_mt to v_mt conversion/Resistance for mt on x-axis ==
  T : Inport  Port=1  LatchInput=off
  Prodct5 : Product  Inputs=*/  RndMeth=Zero
  Product1 : Product  Inputs=3  RndMeth=Zero
  Product3 : Product  Inputs=3  RndMeth=Zero
  Resistivity : Constant  Value=sigma_0_mt
  Resistivity base temperature : Constant  Value=T_0_mt
  Resistivity temperature coefficient : Constant  Value=alpha_0_mt
  Sum1 : Sum  Inputs=|+-
  Sum2 : Sum  Inputs=|++
  Windings1 : Constant  Value=n_mt(1)
  Wire cross sectional area : Constant  Value=A_wire_mt
  wire  circumference : Constant  Value=4*sqrt(A_mt(1))
  R(T) : Outport
  wires:
  Resistivity base temperature/1 -> Sum1/2
  Resistivity temperature coefficient/1 -> Product1/2
  Sum1/1 -> Product1/1
  Resistivity/1 -> Product1/3, Sum2/2
  Product1/1 -> Sum2/1
  Sum2/1 -> Product3/1
  wire  circumference/1 -> Product3/2
  Windings1/1 -> Product3/3
  Product3/1 -> Prodct5/1
  Wire cross sectional area/1 -> Prodct5/2
  T/1 -> Sum1/1
  Prodct5/1 -> R(T)/1

== system components_lib/ACS/Controllers/Desaturation controller/m_mt to v_mt conversion/Resistance for mt on y-axis ==
  T : Inport  Port=1  LatchInput=off
  Prodct5 : Product  Inputs=*/  RndMeth=Zero
  Product1 : Product  Inputs=3  RndMeth=Zero
  Product3 : Product  Inputs=3  RndMeth=Zero
  Resistivity : Constant  Value=sigma_0_mt
  Resistivity base temperature : Constant  Value=T_0_mt
  Resistivity temperature coefficient : Constant  Value=alpha_0_mt
  Sum1 : Sum  Inputs=|+-
  Sum2 : Sum  Inputs=|++
  Windings1 : Constant  Value=n_mt(2)
  Wire cross sectional area : Constant  Value=A_wire_mt
  wire  circumference : Constant  Value=4*sqrt(A_mt(2))
  R(T) : Outport
  wires:
  Prodct5/1 -> R(T)/1
  T/1 -> Sum1/1
  Wire cross sectional area/1 -> Prodct5/2
  Product3/1 -> Prodct5/1
  Windings1/1 -> Product3/3
  wire  circumference/1 -> Product3/2
  Sum2/1 -> Product3/1
  Product1/1 -> Sum2/1
  Resistivity/1 -> Sum2/2, Product1/3
  Sum1/1 -> Product1/1
  Resistivity temperature coefficient/1 -> Product1/2
  Resistivity base temperature/1 -> Sum1/2

== system components_lib/ACS/Controllers/Desaturation controller/m_mt to v_mt conversion/Resistance for mt on z-axis ==
  T : Inport  Port=1  LatchInput=off
  Prodct5 : Product  Inputs=*/  RndMeth=Zero
  Product1 : Product  Inputs=3  RndMeth=Zero
  Product3 : Product  Inputs=3  RndMeth=Zero
  Resistivity : Constant  Value=sigma_0_mt
  Resistivity base temperature : Constant  Value=T_0_mt
  Resistivity temperature coefficient : Constant  Value=alpha_0_mt
  Sum1 : Sum  Inputs=|+-
  Sum2 : Sum  Inputs=|++
  Windings1 : Constant  Value=n_mt(3)
  Wire cross sectional area : Constant  Value=A_wire_mt
  wire  circumference : Constant  Value=4*sqrt(A_mt(3))
  R(T) : Outport
  wires:
  Resistivity base temperature/1 -> Sum1/2
  Resistivity temperature coefficient/1 -> Product1/2
  Sum1/1 -> Product1/1
  Resistivity/1 -> Product1/3, Sum2/2
  Product1/1 -> Sum2/1
  Sum2/1 -> Product3/1
  wire  circumference/1 -> Product3/2
  Windings1/1 -> Product3/3
  Product3/1 -> Prodct5/1
  Wire cross sectional area/1 -> Prodct5/2
  T/1 -> Sum1/1
  Prodct5/1 -> R(T)/1

== system components_lib/ACS/Controllers/Desaturation controller/m_mt to v_mt conversion/electromechanis transfer funtion for mt_x ==
  i_mt : Inport  Port=1  LatchInput=off
  R(T) : Inport  Port=2  LatchInput=off
  Derivative : Derivative
  Gain : Gain  Gain=L_mt(1)
  Product1 : Product  RndMeth=Zero
  Scope : Scope  NumInputPorts=3
      settings: YMin=-5~-5~-5  YMax=5~5~5  SaveName=ScopeData9
  Sum : Sum  Inputs=++|
  v_mt : Outport
  wires:
  Derivative/1 -> Gain/1, Scope/1
  Sum/1 -> v_mt/1, Scope/3
  i_mt/1 -> Derivative/1, Product1/1
  R(T)/1 -> Product1/2, Scope/2
  Product1/1 -> Sum/2
  Gain/1 -> Sum/1

== system components_lib/ACS/Controllers/Desaturation controller/m_mt to v_mt conversion/electromechanis transfer funtion for mt_y  ==
  i_mt : Inport  Port=1  LatchInput=off
  R(T) : Inport  Port=2  LatchInput=off
  Derivative : Derivative
  Gain : Gain  Gain=L_mt(2)
  Product1 : Product  RndMeth=Zero
  Sum : Sum  Inputs=++|
  v_mt : Outport
  wires:
  Gain/1 -> Sum/1
  Product1/1 -> Sum/2
  R(T)/1 -> Product1/2
  i_mt/1 -> Product1/1, Derivative/1
  Sum/1 -> v_mt/1
  Derivative/1 -> Gain/1

== system components_lib/ACS/Controllers/Desaturation controller/m_mt to v_mt conversion/electromechanis transfer funtion for mt_z  ==
  i_mt : Inport  Port=1  LatchInput=off
  R(T) : Inport  Port=2  LatchInput=off
  Derivative : Derivative
  Gain : Gain  Gain=L_mt(3)
  Product1 : Product  RndMeth=Zero
  Sum : Sum  Inputs=++|
  v_mt : Outport
  wires:
  Derivative/1 -> Gain/1
  Sum/1 -> v_mt/1
  i_mt/1 -> Derivative/1, Product1/1
  R(T)/1 -> Product1/2
  Product1/1 -> Sum/2
  Gain/1 -> Sum/1

== system components_lib/ACS/Controllers/Detumble controller/Discrete B-dot controller/Subsystem1 ==
  In1 : Inport  Port=1  LatchInput=off
  Action Port : ActionPort  InitializeStates=reset
  Out1 : Outport  OutputWhenDisabled=reset  InitialOutput=[0 0 0]
  wires:
  In1/1 -> Out1/1

== system components_lib/ACS/Controllers/Detumble controller/Discrete B-dot controller/Subsystem2 ==
  In1 : Inport  Port=1  LatchInput=off
  Action Port : ActionPort  InitializeStates=reset
  Out1 : Outport  OutputWhenDisabled=reset  InitialOutput=[0 0 0]
  wires:
  In1/1 -> Out1/1

== system components_lib/ACS/Controllers/Detumble controller/Discrete B-dot controller/Subsystem3 ==
  In1 : Inport  Port=1  LatchInput=off
  Action Port : ActionPort  InitializeStates=reset
  Out1 : Outport  OutputWhenDisabled=reset  InitialOutput=[0 0 0]
  wires:
  In1/1 -> Out1/1

== system components_lib/ADS/On-board model/ADS on-board models/Albedo model onboard/cos dependent albedo ==
  note: Projection onto
      | the zenith vector
  "Earth -> Sun vector (ECEF)" : Inport  Port=1  LatchInput=off
  Zenith vector (ECEF) : Inport  Port=2  LatchInput=off
  Enable : EnablePort  StatesWhenEnabling=reset
  Abs : Abs
  Dot Product : simulink/Math Operations/Dot Product  InputSameDT=on  OutDataType=sfix(16)  OutScaling=2^-10  DoSatur=off
  Mean solar flux (1366.9 [W/m^2]) : Constant  Value=sun_flux
  Product : Product  RndMeth=Zero
  Product1 : Product  RndMeth=Zero
  Product2 : Product  RndMeth=Zero
  Sun vector  to unit vector : components_lib/Math utilities/Vector operations/to unit vector
  Zentih vector to unit vector : components_lib/Math utilities/Vector operations/to unit vector
  "zenith2ref(u, mrm)" : MATLABFcn  MATLABFcn=zenith2ref(u, mrm)*2
  Albedo vector (I) : Outport
  wires:
  Product2/1 -> Albedo vector (I)/1
  Product1/1 -> Product2/1
  Abs/1 -> Product1/1
  Dot Product/1 -> Abs/1
  Sun vector  to unit vector/1 -> Product/1
  Mean solar flux (1366.9 [W/m^2])/1 -> Product/2
  Product/1 -> Dot Product/1
  "zenith2ref(u, mrm)"/1 -> Product1/2
  Zentih vector to unit vector/1 -> Product2/2, "zenith2ref(u, mrm)"/1, Dot Product/2
  "Earth -> Sun vector (ECEF)"/1 -> Sun vector  to unit vector/1
  Zenith vector (ECEF)/1 -> Zentih vector to unit vector/1

== system components_lib/ADS/On-board model/ADS on-board models/Albedo model onboard/fov matrix albedo ==
  Zenith vector (ECEF) : Inport  Port=1  LatchInput=off
  "Earth -> Sun vector (ECEF)" : Inport  Port=2  LatchInput=off
  q(I->S) : Inport  Port=3  LatchInput=off
  q(I->E) : Inport  Port=4  LatchInput=off
  Enable : EnablePort  StatesWhenEnabling=reset
  Albedo projection : components_lib/ADS/On-board Sensor model/Albedo projection
  Demux : Demux  Outputs=2
  Earth Albedo Model : Subsystem  TreatAsAtomicUnit=on  mask(Earth Albedo Model){eprdata=load('lib/albedo_toolbox/epr_data/2003/ga030101-031231'), redfac=10, Ts=1, enable=on}
      mask prompts: eprdata "Reflectivity Data (EPR Struct):"; redfac "Reduction factor:"; Ts "Sample Time (-1 for inherited):"
      mask help: Calculate Earth Albedo using static data from the EP/TOMS spacecraft.
      mask init:
      | global sy;
      | global sx;
      | sy = round(180/redfac);
      | sx = round(288/redfac);
      mask Help:
      | <b>Input</b><br>
      | Sat: Vector to satellite in ECEF [m]<br>
      | Sun: Vector to the Sun in ECEF [m]<p>
      | <b>Parameters</b><br>
      | Reflectivity Data (EPR Struct): TOMS Reflectivity data [E.U].<br>
      | Reduction factor: Reduce data resolution by this factor.<br>
      | Sample Time (-1 for inherited): Sample Time [s]. The block cannot inherit continuous sample time.<br>
      | Enable: Enable or disable albedo calculation<p>
      | <b>Output</b><br>
      | Albedo: Fraction of solar irradiance received on the satellite. The incoming solar irradiance is 1366.5 W/m^2<p>
      mask CallbackString: |||enable = strcmp(get_param(gcb,'enable'),'on');
      mask Display:
      | image(imread('private/albedoicon.png'));
      | port_label('output', 1, 'Albedo');
      | port_label('input', 1, 'Sat');
      | port_label('input', 2, 'Sun');
  Quaternion inverter1 : components_lib/Math utilities/Quaternion operations/Quaternion inverter
  Rotation of q1 by q2 : components_lib/Math utilities/Quaternion operations/Rotation of q1 by q2
  Sum : Sum  Inputs=|+-
  Vector rotation by q4 : components_lib/Math utilities/Quaternion operations/Vector rotation by q
  "Zenith to nadir " : Gain  Gain=-1
  Albedo vector (I) : Outport
  wires:
  "Earth -> Sun vector (ECEF)"/1 -> Earth Albedo Model/2(r_sun_ecef)
  Zenith vector (ECEF)/1 -> "Zenith to nadir "/1, Earth Albedo Model/1(r_sat_ecef)
  Vector rotation by q4/1 -> Albedo vector (I)/1
  q(I->E)/1 -> Rotation of q1 by q2/2
  q(I->S)/1 -> Quaternion inverter1/1
  Earth Albedo Model/1(a) -> Albedo projection/1
  "Zenith to nadir "/1 -> Albedo projection/2
  Quaternion inverter1/1 -> Rotation of q1 by q2/1, Vector rotation by q4/1
  Rotation of q1 by q2/1 -> Albedo projection/3
  Albedo projection/1 -> Demux/1
  Demux/1 -> Sum/1
  Demux/2 -> Sum/2
  Sum/1 -> Vector rotation by q4/2

== system components_lib/ADS/On-board model/Albedo model onboard/fov matrix albedo/Earth Albedo Model ==
  r_sat_ecef : Inport  Port=1  SampleTime=Ts  LatchInput=off
  r_sun_ecef : Inport  Port=2  SampleTime=Ts  LatchInput=off
  Albedo : Subsystem
  On : Constant  Orientation=down  Value=enable
  Zero-Order Hold1 : ZeroOrderHold  SampleTime=Ts
  Zero-Order Hold2 : ZeroOrderHold  SampleTime=Ts
  a : Outport
  wires:
  Zero-Order Hold1/1 -> Albedo/2(r_sun_ecef)
  Zero-Order Hold2/1 -> Albedo/1(r_sat_ecef)
  r_sun_ecef/1 -> Zero-Order Hold1/1
  Albedo/1(a) -> a/1
  r_sat_ecef/1 -> Zero-Order Hold2/1
  On/1 -> Albedo/Enable

== system components_lib/ADS/On-board model/Orbit and Magnetic field models/TLE and time initialization1/Create TLE and JD ==
  Enable : EnablePort
  Constant : Constant  Value=JulianDay
  "Constant " : Constant  Value=[JulianDay,xndt2o,xndd6o,0,bstar,0,xincl,xnodeo,eo,omegao,xmo,xno]
  Init JD : Outport
  "TLE " : Outport  Port=2
  wires:
  Constant/1 -> Init JD/1
  "Constant "/1 -> "TLE "/1

== system components_lib/ADS/On-board model/Orbit and Magnetic field models/TLE and time initialization3/Create TLE and JD ==
  Enable : EnablePort
  Constant : Constant  Value=JulianDay
  "Constant " : Constant  Value=[JulianDay,xndt2o,xndd6o,0,bstar,0,xincl,xnodeo,eo,omegao,xmo,xno]
  Init JD : Outport
  "TLE " : Outport  Port=2
  wires:
  Constant/1 -> Init JD/1
  "Constant "/1 -> "TLE "/1

== system components_lib/Orbit and Ephemeris/Orbit and Magnetic field models/SGP4 position/TLE and time initialization1/Create TLE and JD ==
  Enable : EnablePort
  Constant : Constant  Value=JulianDay
  "Constant " : Constant  Value=[JulianDay,xndt2o,xndd6o,0,bstar,0,xincl,xnodeo,eo,omegao,xmo,xno]
  Init JD : Outport
  "TLE " : Outport  Port=2
  wires:
  Constant/1 -> Init JD/1
  "Constant "/1 -> "TLE "/1

== system components_lib/Orbit and Ephemeris/Orbit and Magnetic field models/SGP4 position/TLE and time initialization2/Create TLE and JD ==
  Enable : EnablePort
  Constant : Constant  Value=JulianDay
  "Constant " : Constant  Value=[JulianDay,xndt2o,xndd6o,0,bstar,0,xincl,xnodeo,eo,omegao,xmo,xno]
  Init JD : Outport
  "TLE " : Outport  Port=2
  wires:
  "Constant "/1 -> "TLE "/1
  Constant/1 -> Init JD/1

== system components_lib/Sensor Emulation/Emulation of magnetometer/magnetometer sensor block/Vector rotation by q1/Quaternion inverter ==
  q : Inport  Port=1  LatchInput=off
  Demux : Demux
  Demux1 : Demux  Outputs=3
  Gain : Gain  Gain=-1  SaturateOnIntegerOverflow=on
  Mux : Mux
  Mux1 : Mux  Inputs=3
  q^-1 : Outport
  wires:
  Gain/1 -> Demux1/1
  Demux1/3 -> Mux/3
  Demux1/2 -> Mux/2
  Demux1/1 -> Mux/1
  Mux1/1 -> Gain/1
  Demux/3 -> Mux1/3
  Demux/2 -> Mux1/2
  Demux/1 -> Mux1/1
  Demux/4 -> Mux/4
  Mux/1 -> q^-1/1
  q/1 -> Demux/1
